simulink model "comp_offset"  (R2018b)
settings: Solver=VariableStepAuto  StartTime=0.0  StopTime=10.0  RelTol=1e-3
libraries: simulink x1
settings Model: Creator=iamcy  LastModifiedBy=iamcy

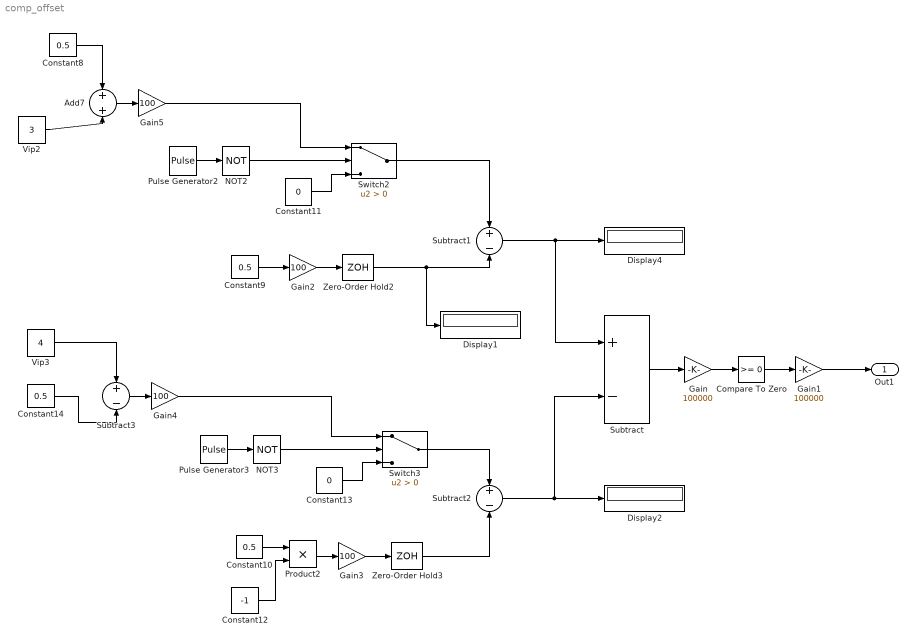
== system comp_offset ==
  Add7 : Sum  Inputs=2
  Compare To Zero : simulink/Logic and Bit Operations/Compare To Zero  relop=>=  OutDataTypeStr=boolean
  Constant{8..10,14} (4 alike) : Constant  Value=0.5
  Constant11 : Constant  Value=0
  Constant12 : Constant  Value=-1
  Constant13 : Constant  Value=0
  Display1 : Display
  Display2 : Display
  Display4 : Display
  Gain : Gain  Gain=100000
  Gain1 : Gain  Gain=100000
  Gain{2..5} (4 alike) : Gain  Gain=100
  NOT2 : Logic  Operator=NOT  IconShape=distinctive  AllPortsSameDT=off  OutDataTypeStr=boolean
  NOT3 : Logic  Operator=NOT  IconShape=distinctive  AllPortsSameDT=off  OutDataTypeStr=boolean
  Product2 : Product
  Pulse Generator2 : DiscretePulseGenerator  PulseType=Time based  Period=13  PulseWidth=100/13
  Pulse Generator3 : DiscretePulseGenerator  PulseType=Time based  Period=13  PulseWidth=100/13
  Subtract{,1..3} (4 alike) : Sum  Inputs=+-
  Switch2 : Switch  Criteria=u2 > Threshold
  Switch3 : Switch  Criteria=u2 > Threshold
  Vip2 : Constant  Value=3
  Vip3 : Constant  Value=4
  Zero-Order Hold2 : ZeroOrderHold  SampleTime=-1
  Zero-Order Hold3 : ZeroOrderHold  SampleTime=-1
  Out1 : Outport
  wires:
  Subtract/1 -> Gain/1
  Gain1/1 -> Out1/1
  Compare To Zero/1 -> Gain1/1
  Gain/1 -> Compare To Zero/1
  Subtract1/1 -> Display4/1, Subtract/1
  Subtract2/1 -> Display2/1, Subtract/2
  Constant9/1 -> Gain2/1
  Constant11/1 -> Switch2/3
  NOT2/1 -> Switch2/2
  Pulse Generator2/1 -> NOT2/1
  Vip2/1 -> Add7/2
  Gain2/1 -> Zero-Order Hold2/1
  Zero-Order Hold2/1 -> Display1/1, Subtract1/2
  Constant8/1 -> Add7/1
  Switch2/1 -> Subtract1/1
  Gain3/1 -> Zero-Order Hold3/1
  Zero-Order Hold3/1 -> Subtract2/2
  Constant10/1 -> Product2/1
  Constant12/1 -> Product2/2
  Product2/1 -> Gain3/1
  NOT3/1 -> Switch3/2
  Pulse Generator3/1 -> NOT3/1
  Constant13/1 -> Switch3/3
  Vip3/1 -> Subtract3/1
  Constant14/1 -> Subtract3/2
  Switch3/1 -> Subtract2/1
  Subtract3/1 -> Gain4/1
  Gain4/1 -> Switch3/1
  Add7/1 -> Gain5/1
  Gain5/1 -> Switch2/1
